simulink model "bramBurst_TransposeMatrix"  (R2021a)
settings: Solver=FixedStepDiscrete  StartTime=0.0  StopTime=44550*Ts  RelTol=1e-3
InitFcn:
  | matched_filter_fft_hdl_init;
model workspace (MAT data in the model file):
  mwTaskManagerKernelLatency = 0
  socvcb = containers.Map
  socvcb.serialization.keys = {12.0018310547, 12.001953125, 12.0020751953, 13.0018310547, 13.001953125, 13.0020751953, 14.0018310547, 14.0020751953, 15.0018310547, 15.0020751953, 15.0133056641, 15.0135498047, 15.0145263672, 15.0153808594, 15.015625, 16.0091552734, 16.0113525391, 16.0115966797, 16.0118408203, 16.0128173828, 16.013671875, 16.0139160156, 16.0141601562, 17.0096435547, 17.0118408203, 17.0146484375, 18.0001220703, 18.0006103516, 19.0001220703, 19.0006103516, 19.0021972656, 19.0023193359, 20.0007324219, 20.0008544922, 30.0006103516, 31.0006103516, 34.0014648438, 35.0014648438, 74.0001220703, 74.0092773438, 74.0178222656, 75.0001220703, 75.0092773438, 75.0178222656, 16098.003418, 20393.0119629, 20461.0002441, 20462.0002441, 21004.0001221, 22191.0001221, 27939.0002441, 29126.0004883, 35663.0014648, 36970.0019531, 48183.0001221, 49370.0001221}
  socvcb.serialization.values : function handle (value not decoded)
  socvcb.serialization.uniformity = 0
  socvcb.serialization.keyType = 'double'
  socvcb.serialization.valueType = 'any'
undefined symbols (not defined in the file or in its folder): columnWindowFun, DTsig_in, DTWindowFun, hdlbramBurst, N1, N2, radarDataCube, Ts
libraries: hdlsllib x35, simulink x11, dsphdlxfrm x1, dsphdlfiltering x1
(part 1 of 2)
settings Model: DataTypeOverride=Off  ExtModeTrigDuration=1  Creator=skuznick  LastModifiedBy=tmealey
settings SolverCC: AlgebraicLoopSolver=TrustRegion  PositivePriorityOrder=on
settings DataIOCC: LimitDataPoints=on  SaveOutput=off  DSMLogging=off  InspectSignalLogs=on  VisualizeSimOutput=off  SaveTime=off
settings OptimizationCC: BlockReduction=off  ConditionallyExecuteInputs=off  DefaultParameterBehavior=Inlined  DefaultUnderspecifiedDataType=single  EnhancedBackFolding=on  PassReuseOutputArgsThreshold=0  EfficientFloat2IntCast=on  MaxStackSize=64  SimCompilerOptimization=on  OptimizeBlockOrder=speed  DifferentSizesBufferReuse=on  OptimizationCustomize=off
settings DebuggingCC: AlgebraicLoopMsg=error  SingleTaskRateTransMsg=error  ParameterPrecisionLossMsg=none  ParameterTunabilityLossMsg=error  FixptConstUnderflowMsg=warning  FixptConstOverflowMsg=warning  AllowSymbolicDim=off  PregeneratedLibrarySubsystemCodeDiagnostic=none  SFUnexpectedBacktrackingDiag=warning  SFNoUnconditionalDefaultTransitionDiag=warning  SFExecutionAtInitializationDiag=none  SFMachineParentedDataDiag=warning  IntegerSaturationMsg=none  ArithmeticOperatorsInVariantConditions=warning
settings HardwareCC: TargetBitPerPointer=64  TargetBitPerSizeT=64  TargetBitPerPtrDiffT=64  TargetLongLongMode=on  TargetIntDivRoundTo=Zero  TargetEndianess=LittleEndian  TargetWordSize=64  TargetHWDeviceType=Custom Processor->MATLAB Host Computer  ProdEqTarget=off  HardwareBoardFeatureSet=SoCBlockset
settings SFSimCC: SimUseLocalCustomCode=off  MATLABDynamicMemAlloc=off  CustomCodeUndefinedFunction=UseInterfaceOnly
settings RTWCC: Description=Generic Real-Time Target  GenerateReport=on  RTWUseLocalCustomCode=off  LaunchReport=on
settings CodeAppCC: ForceParamTrailComments=on  OperatorAnnotations=on
settings GRTTargetCC: TargetLangStandard=C89/C90 (ANSI)
settings ConfigComp: CovMetricSettings=dw  CovSaveCumulativeToWorkspaceVar=on  CovSaveSingleToWorkspaceVar=on  CovExternalEMLEnable=off  CovSFcnEnable=off

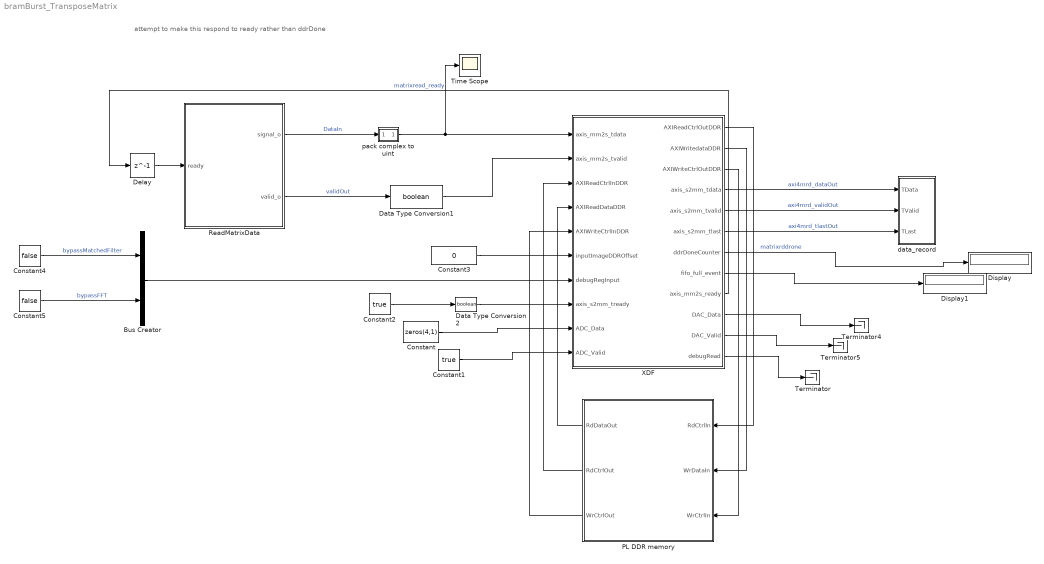
== system bramBurst_TransposeMatrix ==
  note: attempt to make this respond to ready rather than ddrDone
  Bus Creator : BusCreator  Inputs=2
  Constant : Constant  Value=zeros(4,1)  OutDataTypeStr=int16  SampleTime=-1
  Constant1 : Constant  Value=true  OutDataTypeStr=boolean  SampleTime=-1
  Constant2 : Constant  Value=true  SampleTime=-1
  Constant3 : Constant  Value=0  OutDataTypeStr=uint32  SampleTime=-1
  Constant4 : Constant  Value=false  SampleTime=-1
  Constant5 : Constant  Value=false  SampleTime=-1
  Data Type Conversion1 : DataTypeConversion  OutDataTypeStr=boolean
  Data Type Conversion2 : DataTypeConversion  OutDataTypeStr=boolean
  Delay : Delay  DelayLength=1
  Display : Display
  Display1 : Display
  PL DDR memory : Subsystem
  ReadMatrixData : MATLAB Function  TreatAsAtomicUnit=on  SystemSampleTime=Ts  mask{MatrixInput=radarDataCube, ValidGap=0, GapsInMatrix=40, Ts=Ts}
      mask prompts: MatrixInput "Matrix value"; ValidGap "Valid Gap between columns"; GapsInMatrix "Valid Gap between matrix writes"; Ts "Sample Time"
  Terminator : Terminator
  Terminator4 : Terminator
  Terminator5 : Terminator
  Time Scope : Scope
  XDF : Subsystem  TreatAsAtomicUnit=on
  "data_record " : Subsystem
  pack complex to uint : Subsystem
  wires:
  PL DDR memory/2(RdCtrlOut) -> XDF/3(AXIReadCtrlInDDR)
  PL DDR memory/3(WrCtrlOut) -> XDF/5(AXIWriteCtrlInDDR)
  PL DDR memory/1(RdDataOut) -> XDF/4(AXIReadDataDDR)
  XDF/1(AXIReadCtrlOutDDR) -> PL DDR memory/1(RdCtrlIn)
  XDF/2(AXIWritedataDDR) -> PL DDR memory/2(WrDataIn)
  XDF/3(AXIWriteCtrlOutDDR) -> PL DDR memory/3(WrCtrlIn)
  Constant3/1 -> XDF/6(inputImageDDROffset)
  ReadMatrixData/1(signal_o) -> pack complex to uint/1(In1)  "DataIn"
  ReadMatrixData/2(valid_o) -> Data Type Conversion1/1  "validOut"
  pack complex to uint/1(Out1) -> Time Scope/1, XDF/1(axis_mm2s_tdata)
  XDF/4(axis_s2mm_tdata) -> "data_record "/1(TData)  "axi4mrd_dataOut"
  XDF/5(axis_s2mm_tvalid) -> "data_record "/2(TValid)  "axi4mrd_validOut"
  Data Type Conversion1/1 -> XDF/2(axis_mm2s_tvalid)
  XDF/8(fifo_full_event) -> Display1/1
  XDF/7(ddrDoneCounter) -> Display/1  "matrixrddrone"
  XDF/9(axis_mm2s_ready) -> Delay/1  "matrixread_ready"
  Constant/1 -> XDF/9(ADC_Data)
  Constant1/1 -> XDF/10(ADC_Valid)
  XDF/10(DAC_Data) -> Terminator4/1
  XDF/11(DAC_Valid) -> Terminator5/1
  Data Type Conversion2/1 -> XDF/8(axis_s2mm_tready)
  XDF/6(axis_s2mm_tlast) -> "data_record "/3(TLast)  "axi4mrd_tlastOut"
  Constant2/1 -> Data Type Conversion2/1
  Delay/1 -> ReadMatrixData/1(ready)
  Constant4/1 -> Bus Creator/1  "bypassMatchedFilter"
  Constant5/1 -> Bus Creator/2  "bypassFFT"
  Bus Creator/1 -> XDF/7(debugRegInput)
  XDF/12(debugRead) -> Terminator/1

== system bramBurst_TransposeMatrix/PL DDR memory ==
  RdCtrlIn : Inport
  WrDataIn : Inport  Port=2
  WrCtrlIn : Inport  Port=3
  DDR : Subsystem  mask{DDR_SIZE=N1*N2*4*4, INTERFACE_WORD_LENGTH_SELECT=64, INTERFACE_NUM_WORDS=1, INIT_DATA=uint32(1:100), INIT_ADDR=0, BANDWIDTH_DERATING_PCT=10, READ_DOWNTIME=4, toggle=off, save=on, varnameStr='sim_ddr_data'}
      mask prompts: DDR_SIZE "Memory size (bytes):"; INTERFACE_WORD_LENGTH_SELECT "Word length (bits):"; INTERFACE_NUM_WORDS "Number of words:"; INIT_DATA "Initialization data:"; INIT_ADDR "Starting address:"; BANDWIDTH_DERATING_PCT "Bandwidth derating (%)"; READ_DOWNTIME "Read burst downtime (cycles)"; toggle "Read valid toggling"; save "Enabled"; varnameStr "Variable name:"
      mask help: DDR Simulation model
      mask init:
      | blkH = gcbh;
      | 
      | if(DDR_SIZE<=0)
      |     error('Specify a positive value for memory size.' )  
      | end
      | 
      | if( (BANDWIDTH_DERATING_PCT<0) || (BANDWIDTH_DERATING_PCT > 100) )
      |   error('Specify bandwidth derating as a percentage 0-100.' )  
      | end
      | 
      | if (INIT_ADDR < 0)
      |     error('Specify a positive value for starting address.');
      | end
      | 
      | if (mod(INIT_ADDR,4)~=0)
      |     error('Starting address should be multiple of 4 (32-bit aligned).');
      | end
      | 
      | BANDWIDTH_DERATING = BANDWIDTH_DERATING_PCT/100;
      | 
      | INTERFACE_WORD_LENGTH = str2double(get_param(blkH,'INTERFACE_WORD_LENGTH_SELECT'));
      | 
      | DATA_NUM_BYTES = INTERFACE_WORD_LENGTH/8 * INTERFACE_NUM_WORDS;
      | ADDR_BIT_SHIFT = nextpow2(DATA_NUM_BYTES);
      | 
      | switch INTERFACE_WORD_LENGTH
      |     case {8, 16, 32}
      |         INTERFACE_DT = sprintf('uint%d',INTERFACE_WORD_LENGTH);
      |     case {64, 128}
      |         INTERFACE_DT = numerictype(0,INTERFACE_WORD_LENGTH,0);
      | end
      mask TypeOptions INTERFACE_WORD_LENGTH_SELECT: 8 | 16 | 32 | 64 | 128
      mask Callback INTERFACE_WORD_LENGTH_SELECT:
      | blkH = gcbh;
      | mObj  = Simulink.Mask.get(blkH);
      | txtObj = mObj.getDialogControl('INTERFACE_WIDTH_TEXT');
      | 
      | wordLength = str2double(get_param(blkH,'INTERFACE_WORD_LENGTH_SELECT'));
      | numWords = str2double(get_param(blkH,'INTERFACE_NUM_WORDS'));
      | 
      | if isnan(numWords)
      |     valStr = '';
      | else
      |     valStr = num2str(wordLength*numWords);
      | end
      | 
      | txt = sprintf('Total word length:  %s',valStr);
      | 
      | txtObj.Prompt = txt;
      mask Callback INTERFACE_NUM_WORDS:
      | blkH = gcbh;
      | mObj  = Simulink.Mask.get(blkH);
      | txtObj = mObj.getDialogControl('INTERFACE_WIDTH_TEXT');
      | 
      | wordLength = str2double(get_param(blkH,'INTERFACE_WORD_LENGTH_SELECT'));
      | numWords = str2double(get_param(blkH,'INTERFACE_NUM_WORDS'));
      | 
      | if isnan(numWords)
      |     valStr = '';
      | else
      |     valStr = num2str(wordLength*numWords);
      | end
      | 
      | txt = sprintf('Total word length:  %s',valStr);
      | 
      | txtObj.Prompt = txt;
      mask TypeOptions save: Write DDR Data to Workspace/Save to Workspace/save
      mask TypeOptions varnameStr: Write DDR Data to Workspace/Save to Workspace/varnameStr
      mask DialogControl DescGroupVar Prompt: DDR
      mask DialogControl Container6 Prompt: Interface
      mask DialogControl INTERFACE_WIDTH_TEXT Prompt: Total word length:  64
      mask DialogControl DDR_INIT Prompt: Initialization
      mask DialogControl Container7 Prompt: Behavioral
      mask DialogControl BANDWIDTH_DERATING_PCT Tooltip: between 0 to 1
      mask DialogControl Container5 Prompt: Save memory contents at end of simulation
  RdDataOut : Outport  VectorParamsAs1DForOutWhenUnconnected=off
  RdCtrlOut : Outport  Port=2  VectorParamsAs1DForOutWhenUnconnected=off
  WrCtrlOut : Outport  Port=3  VectorParamsAs1DForOutWhenUnconnected=off
  wires:
  WrDataIn/1 -> DDR/2(axi_wr_data)
  RdCtrlIn/1 -> DDR/1(axi_rd_m2s)
  DDR/1(axi_rd_data) -> RdDataOut/1
  DDR/2(axi_rd_s2m) -> RdCtrlOut/1
  WrCtrlIn/1 -> DDR/3(axi_wr_m2s)
  DDR/3(axi_wr_s2m) -> WrCtrlOut/1

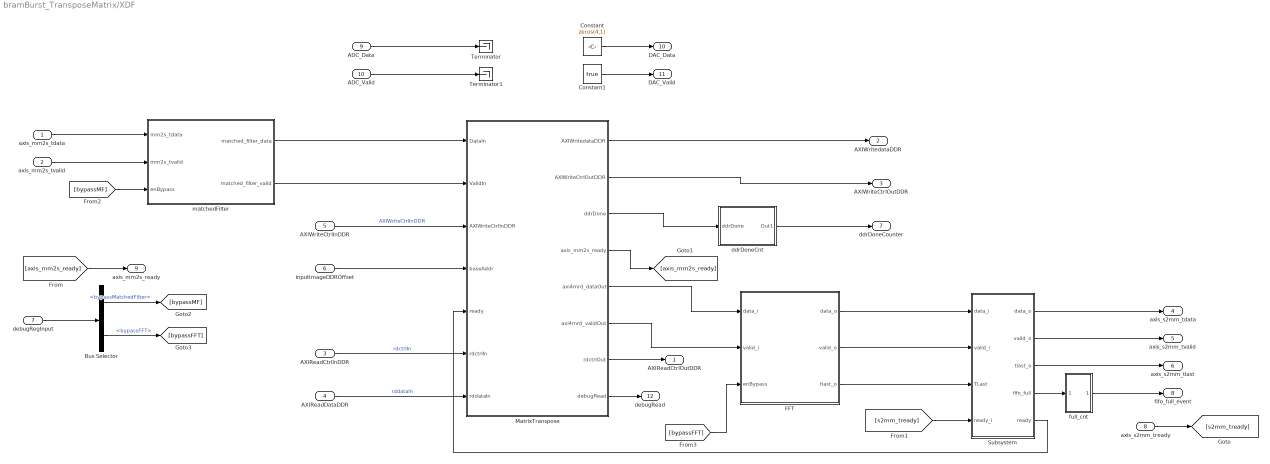
== system bramBurst_TransposeMatrix/XDF ==
  axis_mm2s_tdata : Inport
  axis_mm2s_tvalid : Inport  Port=2
  AXIReadCtrlInDDR : Inport  Port=3
  AXIReadDataDDR : Inport  Port=4
  AXIWriteCtrlInDDR : Inport  Port=5
  inputImageDDROffset : Inport  Port=6
  debugRegInput : Inport  Port=7
  axis_s2mm_tready : Inport  Port=8
  ADC_Data : Inport  Port=9
  ADC_Valid : Inport  Port=10
  Bus Selector : BusSelector  OutputSignals=bypassMatchedFilter,bypassFFT
  Constant : Constant  Value=zeros(4,1)  OutDataTypeStr=int16  SampleTime=-1
  Constant1 : Constant  Value=true  OutDataTypeStr=boolean  SampleTime=-1
  FFT : Subsystem
  MatrixTranspose : Subsystem
  Subsystem : Subsystem
  Terminator : Terminator
  Terminator1 : Terminator
  ddrDoneCnt : Subsystem
  full_cnt : Subsystem
  matchedFilter : Subsystem
  AXIReadCtrlOutDDR : Outport  VectorParamsAs1DForOutWhenUnconnected=off
  AXIWritedataDDR : Outport  Port=2  VectorParamsAs1DForOutWhenUnconnected=off
  AXIWriteCtrlOutDDR : Outport  Port=3  VectorParamsAs1DForOutWhenUnconnected=off
  axis_s2mm_tdata : Outport  Port=4  VectorParamsAs1DForOutWhenUnconnected=off
  axis_s2mm_tvalid : Outport  Port=5
  axis_s2mm_tlast : Outport  Port=6
  ddrDoneCounter : Outport  Port=7
  fifo_full_event : Outport  Port=8
  axis_mm2s_ready : Outport  Port=9
  DAC_Data : Outport  Port=10
  DAC_Valid : Outport  Port=11
  debugRead : Outport  Port=12
  wires:
  axis_mm2s_tvalid/1 -> matchedFilter/2(mm2s_tvalid)
  ADC_Data/1 -> Terminator/1
  ADC_Valid/1 -> Terminator1/1
  Constant/1 -> DAC_Data/1
  Constant1/1 -> DAC_Valid/1
  axis_mm2s_tdata/1 -> matchedFilter/1(mm2s_tdata)
  ddrDoneCnt/1(Out1) -> ddrDoneCounter/1
  Subsystem/1(data_o) -> axis_s2mm_tdata/1
  Subsystem/2(valid_o) -> axis_s2mm_tvalid/1
  Subsystem/3(tlast_o) -> axis_s2mm_tlast/1
  full_cnt/1(Out1) -> fifo_full_event/1
  Subsystem/4(fifo_full) -> full_cnt/1(In1)
  FFT/2(valid_o) -> Subsystem/2(valid_i)
  FFT/3(tlast_o) -> Subsystem/3(TLast)
  FFT/1(data_o) -> Subsystem/1(data_i)
  matchedFilter/1(matched_filter_data) -> MatrixTranspose/1(DataIn)
  matchedFilter/2(matched_filter_valid) -> MatrixTranspose/2(ValidIn)
  AXIWriteCtrlInDDR/1 -> MatrixTranspose/3(AXIWriteCtrlInDDR)  "AXIWriteCtrlInDDR"
  inputImageDDROffset/1 -> MatrixTranspose/4(baseAddr)
  Subsystem/5(ready) -> MatrixTranspose/5(ready)
  AXIReadCtrlInDDR/1 -> MatrixTranspose/6(rdctrlIn)  "rdctrlIn"
  AXIReadDataDDR/1 -> MatrixTranspose/7(rddataIn)  "rddataIn"
  MatrixTranspose/1(AXIWritedataDDR) -> AXIWritedataDDR/1
  MatrixTranspose/2(AXIWriteCtrlOutDDR) -> AXIWriteCtrlOutDDR/1
  MatrixTranspose/3(ddrDone) -> ddrDoneCnt/1(ddrDone)
  MatrixTranspose/4(axis_mm2s_ready) -> [axis_mm2s_ready]
  MatrixTranspose/5(axi4mrd_dataOut) -> FFT/1(data_i)
  MatrixTranspose/6(axi4mrd_validOut) -> FFT/2(valid_i)
  MatrixTranspose/7(rdctrlOut) -> AXIReadCtrlOutDDR/1
  [axis_mm2s_ready] -> axis_mm2s_ready/1
  axis_s2mm_tready/1 -> [s2mm_tready]
  [s2mm_tready] -> Subsystem/4(ready_i)
  debugRegInput/1 -> Bus Selector/1
  Bus Selector/1 -> [bypassMF]  "<bypassMatchedFilter>"
  Bus Selector/2 -> [bypassFFT]  "<bypassFFT>"
  [bypassMF] -> matchedFilter/3(enBypass)
  [bypassFFT] -> FFT/3(enBypass)
  MatrixTranspose/8(debugRead) -> debugRead/1

== system bramBurst_TransposeMatrix/data_record  ==
  TData : Inport
  TValid : Inport  Port=2
  TLast : Inport  Port=3
  Compare To Constant : simulink/Logic and Bit Operations/Compare To Constant  relop=>=  const=N1*N2*1  OutDataTypeStr=boolean
  HDL Counter : hdlsllib/Sources/HDL Counter  CountType=Free running  CountInit=0  CountStep=1  CountMax=25  CountFromType=Initial value  CountFrom=0  CountResetPort=off  CountLoadPort=off  CountEnbPort=on  CountDirPort=off  CountHitOutputPort=off  CountDataType=Unsigned  CountWordLen=32  CountFracLen=0  CountSampTime=1
  Stop Simulation : Stop
  To Workspace : ToWorkspace  VariableName=rdMat  SampleTime=-1
      settings: Save2DSignal=2-D array (concatenate along first dimension)
  To Workspace1 : ToWorkspace  VariableName=rdValid  SampleTime=-1
      settings: Save2DSignal=2-D array (concatenate along first dimension)
  To Workspace2 : ToWorkspace  VariableName=rdTlast  SampleTime=-1
      settings: Save2DSignal=2-D array (concatenate along first dimension)
  "unpack uint to complex " : Subsystem
  wires:
  HDL Counter/1 -> Compare To Constant/1
  Compare To Constant/1 -> Stop Simulation/1
  TValid/1 -> HDL Counter/1, To Workspace1/1
  TData/1 -> "unpack uint to complex "/1(TData)
  TLast/1 -> To Workspace2/1
  "unpack uint to complex "/1(Out1) -> To Workspace/1

== system bramBurst_TransposeMatrix/pack complex to uint ==
  In1 : Inport
  Bit Concat : hdlsllib/Logic and Bit Operations/Bit Concat  numInputs=2
  Bit Concat1 : hdlsllib/Logic and Bit Operations/Bit Concat  Commented=on  numInputs=2
  Complex to Real-Imag : ComplexToRealImag
  Complex to Real-Imag1 : ComplexToRealImag  Commented=on
  Data Type Conversion1 : DataTypeConversion  Commented=on  OutDataTypeStr=fixdt(1,32,28)
  Data Type Conversion2 : DataTypeConversion  OutDataTypeStr=DTsig_in
  Data Type Conversion3 : DataTypeConversion  OutDataTypeStr=uint64  ConvertRealWorld=Stored Integer (SI)
  Out1 : Outport
  wires:
  Complex to Real-Imag/2 -> Bit Concat/2
  Data Type Conversion2/1 -> Complex to Real-Imag/1  "Data"
  Complex to Real-Imag/1 -> Bit Concat/1
  In1/1 -> Data Type Conversion1/1, Data Type Conversion2/1
  Data Type Conversion1/1 -> Complex to Real-Imag1/1  "Data"
  Complex to Real-Imag1/1 -> Bit Concat1/1
  Complex to Real-Imag1/2 -> Bit Concat1/2
  Data Type Conversion3/1 -> Out1/1
  Bit Concat/1 -> Data Type Conversion3/1

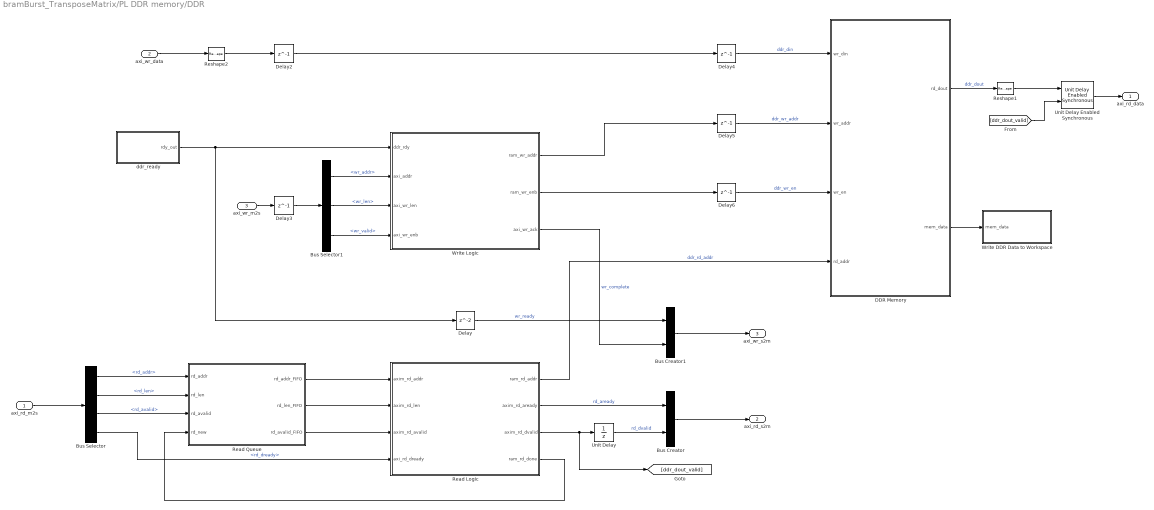
== system bramBurst_TransposeMatrix/PL DDR memory/DDR ==
  axi_rd_m2s : Inport
  axi_wr_data : Inport  Port=2  OutDataTypeStr=INTERFACE_DT  PortDimensions=INTERFACE_NUM_WORDS
  axi_wr_m2s : Inport  Port=3
  Bus Creator : BusCreator  Inputs=2
  Bus Creator1 : BusCreator  Inputs=2  OutDataTypeStr=Bus: BusAXIWriteCtrlS2M  NonVirtualBus=on
  Bus Selector : BusSelector  OutputSignals=rd_addr,rd_len,rd_avalid,rd_dready
  Bus Selector1 : BusSelector  OutputSignals=wr_addr,wr_len,wr_valid
  DDR Memory : MATLAB Function  TreatAsAtomicUnit=on
  Delay : Delay
  Delay{2..6} (5 alike) : Delay  DelayLength=1
  Read Logic : Subsystem
  Read Queue : Subsystem
  Reshape1 : Reshape
  Reshape2 : Reshape
  Unit Delay : UnitDelay  SampleTime=-1  HasFrameUpgradeWarning=on
  Unit Delay Enabled Synchronous : hdlsllib/Discrete/Unit Delay Enabled Synchronous  InitialCondition=0.0  SampleTime=-1
      settings: SourceProductBaseCode=SL
  Write DDR Data to Workspace : Subsystem  TreatAsAtomicUnit=on
  Write Logic : Subsystem
  ddr_ready : Subsystem
  axi_rd_data : Outport  VectorParamsAs1DForOutWhenUnconnected=off
  axi_rd_s2m : Outport  Port=2  VectorParamsAs1DForOutWhenUnconnected=off
  axi_wr_s2m : Outport  Port=3  VectorParamsAs1DForOutWhenUnconnected=off
  wires:
  [ddr_dout_valid] -> Unit Delay Enabled Synchronous/2
  Unit Delay/1 -> Bus Creator/2  "rd_dvalid"
  Unit Delay Enabled Synchronous/1 -> axi_rd_data/1
  Reshape1/1 -> Unit Delay Enabled Synchronous/1
  Reshape2/1 -> Delay2/1
  axi_wr_data/1 -> Reshape2/1
  Read Queue/1(rd_addr_FIFO) -> Read Logic/1(axim_rd_addr)
  Bus Selector/1 -> Read Queue/1(rd_addr)  "<rd_addr>"
  Read Queue/3(rd_avalid_FIFO) -> Read Logic/3(axim_rd_avalid)
  Read Queue/2(rd_len_FIFO) -> Read Logic/2(axim_rd_len)
  Bus Selector/3 -> Read Queue/3(rd_avalid)  "<rd_avalid>"
  Read Logic/4(ram_rd_done) -> Read Queue/4(rd_new)
  Bus Selector/2 -> Read Queue/2(rd_len)  "<rd_len>"
  DDR Memory/2(mem_data) -> Write DDR Data to Workspace/1(mem_data)
  Delay6/1 -> DDR Memory/3(wr_en)  "ddr_wr_en"
  Delay5/1 -> DDR Memory/2(wr_addr)  "ddr_wr_addr"
  Delay4/1 -> DDR Memory/1(wr_din)  "ddr_din"
  axi_rd_m2s/1 -> Bus Selector/1
  Bus Selector/4 -> Read Logic/4(axi_rd_dready)  "<rd_dready>"
  Delay3/1 -> Bus Selector1/1
  Delay2/1 -> Delay4/1
  Delay/1 -> Bus Creator1/1  "wr_ready"
  Write Logic/3(axi_wr_ack) -> Bus Creator1/2  "wr_complete"
  Bus Creator1/1 -> axi_wr_s2m/1
  ddr_ready/1(rdy_out) -> Delay/1, Write Logic/1(ddr_rdy)
  Read Logic/3(axim_rd_dvalid) -> Unit Delay/1, [ddr_dout_valid]
  Bus Creator/1 -> axi_rd_s2m/1
  Read Logic/2(axim_rd_aready) -> Bus Creator/1  "rd_aready"
  Bus Selector1/2 -> Write Logic/3(axi_wr_len)  "<wr_len>"
  Bus Selector1/3 -> Write Logic/4(axi_wr_enb)  "<wr_valid>"
  axi_wr_m2s/1 -> Delay3/1
  Bus Selector1/1 -> Write Logic/2(axi_addr)  "<wr_addr>"
  Write Logic/1(ram_wr_addr) -> Delay5/1
  Read Logic/1(ram_rd_addr) -> DDR Memory/4(rd_addr)  "ddr_rd_addr"
  DDR Memory/1(rd_dout) -> Reshape1/1  "ddr_dout"
  Write Logic/2(ram_wr_enb) -> Delay6/1

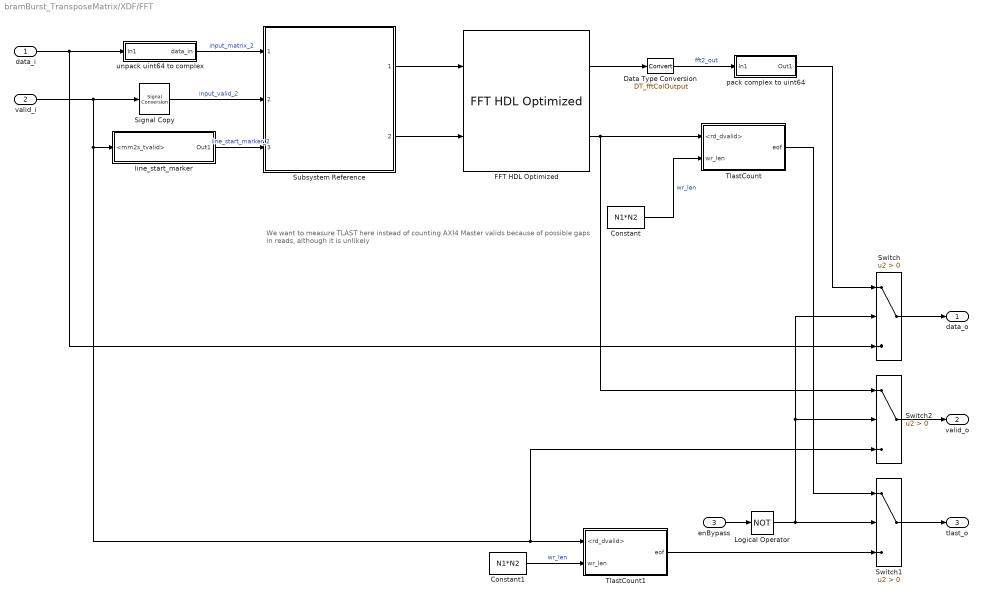
== system bramBurst_TransposeMatrix/XDF/FFT ==
  note: We want to measure TLAST here instead of counting
      | AXI4 Master valids because of possible gaps in reads, although it is unlikely
  data_i : Inport
  valid_i : Inport  Port=2
  enBypass : Inport  Port=3
  Constant : Constant  Value=N1*N2  OutDataTypeStr=uint32  SampleTime=-1
  Constant1 : Constant  Value=N1*N2  OutDataTypeStr=uint32  SampleTime=-1
  Data Type Conversion : DataTypeConversion  OutDataTypeStr=DT_fftColOutput
  FFT HDL Optimized : dsphdlxfrm/FFT HDL Optimized  FFTLength=N2  Architecture=Streaming Radix 2^2  ComplexMultiplication=Use 4 multipliers and 2 adders  BitReversedOutput=off  BitReversedInput=off  Normalize=on  SimulateUsing=Code generation  RoundingMethod=Floor  ResetInputPort=off  StartOutputPort=off  EndOutputPort=off
      settings: SourceProductBaseCode=DS
  Logical Operator : Logic  Operator=NOT  IconShape=distinctive  AllPortsSameDT=off  OutDataTypeStr=boolean
  Signal Copy : SignalConversion  OverrideOpt=off
  Subsystem Reference : Subsystem  ReferencedSubsystem=window_taper  windowFun=fi(columnWindowFun,DTWindowFun)
  Switch : Switch  Criteria=u2 > Threshold
  Switch1 : Switch  Criteria=u2 > Threshold
  Switch2 : Switch  Criteria=u2 > Threshold
  TlastCount : Subsystem
  TlastCount1 : Subsystem
  line_start_marker : Subsystem
  pack complex to uint64 : Subsystem
  "unpack uint64 to complex " : Subsystem
  data_o : Outport
  valid_o : Outport  Port=2
  tlast_o : Outport  Port=3
  wires:
  Data Type Conversion/1 -> pack complex to uint64/1(In1)  "fft2_out"
  Subsystem Reference/2 -> FFT HDL Optimized/2
  Subsystem Reference/1 -> FFT HDL Optimized/1
  "unpack uint64 to complex "/1(data_in) -> Subsystem Reference/1  "input_matrix_2"
  line_start_marker/1(Out1) -> Subsystem Reference/3  "line_start_marker_2"
  FFT HDL Optimized/1 -> Data Type Conversion/1
  Signal Copy/1 -> Subsystem Reference/2  "input_valid_2"
  pack complex to uint64/1(Out1) -> Switch/1
  data_i/1 -> Switch/3, "unpack uint64 to complex "/1(In1)
  enBypass/1 -> Logical Operator/1
  Logical Operator/1 -> Switch2/2, Switch/2, Switch1/2
  Constant/1 -> TlastCount/2(wr_len)  "wr_len"
  FFT HDL Optimized/2 -> TlastCount/1(<rd_dvalid>), Switch2/1
  TlastCount/1(eof) -> Switch1/1
  valid_i/1 -> line_start_marker/1(<mm2s_tvalid>), Switch2/3, TlastCount1/1(<rd_dvalid>), Signal Copy/1
  Constant1/1 -> TlastCount1/2(wr_len)  "wr_len"
  TlastCount1/1(eof) -> Switch1/3
  Switch/1 -> data_o/1
  Switch2/1 -> valid_o/1
  Switch1/1 -> tlast_o/1

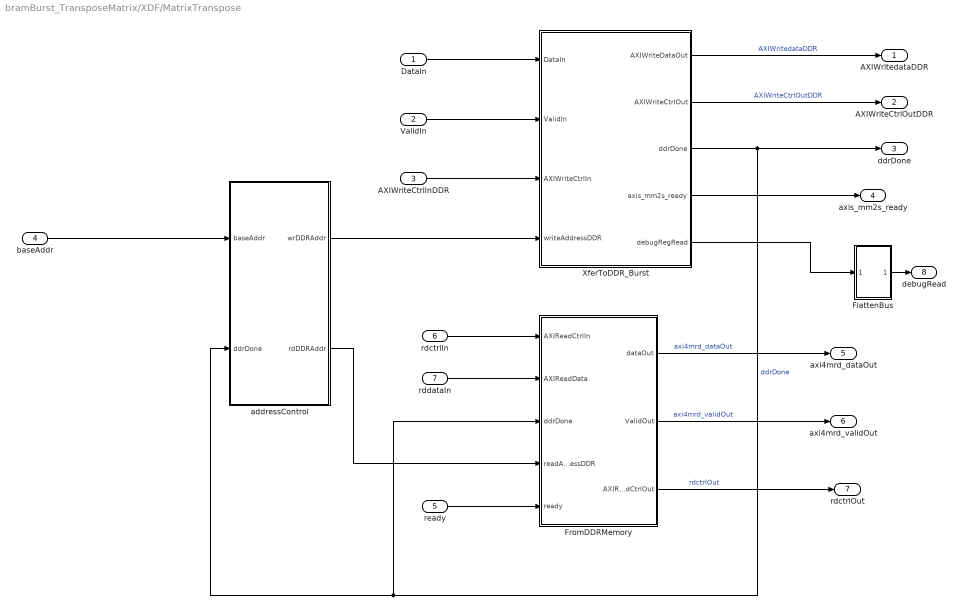
== system bramBurst_TransposeMatrix/XDF/MatrixTranspose ==
  DataIn : Inport
  ValidIn : Inport  Port=2
  AXIWriteCtrlInDDR : Inport  Port=3
  baseAddr : Inport  Port=4
  ready : Inport  Port=5
  rdctrlIn : Inport  Port=6
  rddataIn : Inport  Port=7
  FlattenBus : Subsystem
  FromDDRMemory : Subsystem
  XferToDDR_Burst : Subsystem  VariantControl=XferToDDR_Burst
  addressControl : Subsystem
  AXIWritedataDDR : Outport
  AXIWriteCtrlOutDDR : Outport  Port=2
  ddrDone : Outport  Port=3
  axis_mm2s_ready : Outport  Port=4
  axi4mrd_dataOut : Outport  Port=5
  axi4mrd_validOut : Outport  Port=6
  rdctrlOut : Outport  Port=7
  debugRead : Outport  Port=8
  wires:
  addressControl/2(rdDDRAddr) -> FromDDRMemory/4(readAddressDDR)
  XferToDDR_Burst/3(ddrDone) -> FromDDRMemory/3(ddrDone), addressControl/2(ddrDone), ddrDone/1  "ddrDone"
  FromDDRMemory/1(dataOut) -> axi4mrd_dataOut/1  "axi4mrd_dataOut"
  FromDDRMemory/3(AXIReadCtrlOut) -> rdctrlOut/1  "rdctrlOut"
  addressControl/1(wrDDRAddr) -> XferToDDR_Burst/4(writeAddressDDR)
  DataIn/1 -> XferToDDR_Burst/1(DataIn)
  XferToDDR_Burst/2(AXIWriteCtrlOut) -> AXIWriteCtrlOutDDR/1  "AXIWriteCtrlOutDDR"
  XferToDDR_Burst/1(AXIWriteDataOut) -> AXIWritedataDDR/1  "AXIWritedataDDR"
  rddataIn/1 -> FromDDRMemory/2(AXIReadData)
  XferToDDR_Burst/4(axis_mm2s_ready) -> axis_mm2s_ready/1
  FromDDRMemory/2(ValidOut) -> axi4mrd_validOut/1  "axi4mrd_validOut"
  rdctrlIn/1 -> FromDDRMemory/1(AXIReadCtrlIn)
  baseAddr/1 -> addressControl/1(baseAddr)
  AXIWriteCtrlInDDR/1 -> XferToDDR_Burst/3(AXIWriteCtrlIn)
  ValidIn/1 -> XferToDDR_Burst/2(ValidIn)
  ready/1 -> FromDDRMemory/5(ready)
  XferToDDR_Burst/5(debugRegRead) -> FlattenBus/1(In1)
  FlattenBus/1(Out1) -> debugRead/1

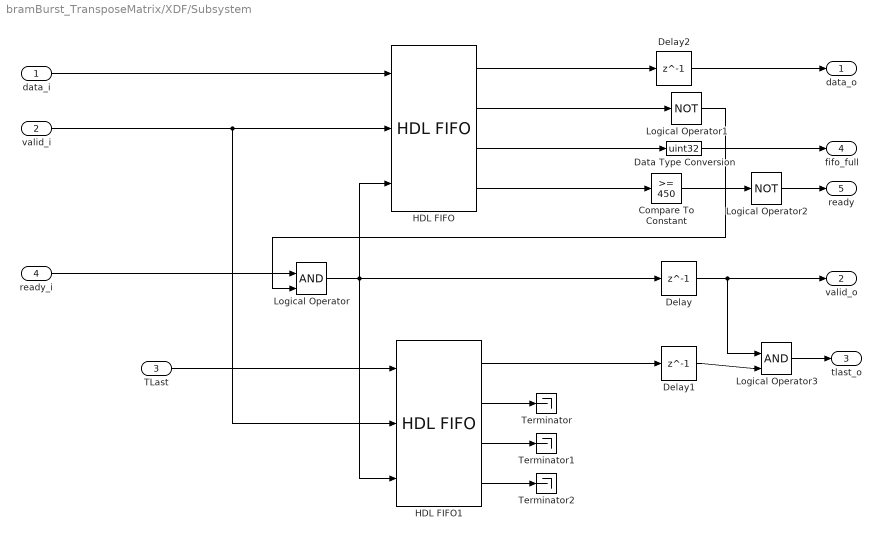
== system bramBurst_TransposeMatrix/XDF/Subsystem ==
  data_i : Inport
  valid_i : Inport  Port=2
  TLast : Inport  Port=3
  ready_i : Inport  Port=4
  Compare To Constant : simulink/Logic and Bit Operations/Compare To Constant  relop=>=  const=450  OutDataTypeStr=boolean
  Data Type Conversion : DataTypeConversion  OutDataTypeStr=uint32
  Delay : Delay  DelayLength=1
  Delay1 : Delay  DelayLength=1
  Delay2 : Delay  DelayLength=1
  HDL FIFO : hdlsllib/HDL RAMs/HDL FIFO  fifo_size=512  mode=FWFT  ratio=1  push_msg=Warning  pop_msg=Warning  show_empty=on  show_full=on  show_num=on  LabelModeActiveChoice_Mode=FWFT
      settings: SourceProductBaseCode=SL
  HDL FIFO1 : hdlsllib/HDL RAMs/HDL FIFO  fifo_size=512  mode=FWFT  ratio=1  push_msg=Warning  pop_msg=Warning  show_empty=on  show_full=on  show_num=on  LabelModeActiveChoice_Mode=FWFT
      settings: SourceProductBaseCode=SL
  Logical Operator : Logic  IconShape=distinctive  AllPortsSameDT=off  OutDataTypeStr=boolean
  Logical Operator1 : Logic  Operator=NOT  IconShape=distinctive  AllPortsSameDT=off  OutDataTypeStr=boolean
  Logical Operator2 : Logic  Operator=NOT  IconShape=distinctive  AllPortsSameDT=off  OutDataTypeStr=boolean
  Logical Operator3 : Logic  IconShape=distinctive  AllPortsSameDT=off  OutDataTypeStr=boolean
  Terminator : Terminator
  Terminator1 : Terminator
  Terminator2 : Terminator
  data_o : Outport
  valid_o : Outport  Port=2
  tlast_o : Outport  Port=3
  fifo_full : Outport  Port=4
  ready : Outport  Port=5
  wires:
  valid_i/1 -> HDL FIFO1/2, HDL FIFO/2
  Logical Operator1/1 -> Logical Operator/2
  HDL FIFO/4 -> Compare To Constant/1
  HDL FIFO/1 -> Delay2/1
  Logical Operator/1 -> HDL FIFO1/3, Delay/1, HDL FIFO/3
  HDL FIFO/3 -> Data Type Conversion/1
  Delay2/1 -> data_o/1
  HDL FIFO/2 -> Logical Operator1/1
  data_i/1 -> HDL FIFO/1
  Data Type Conversion/1 -> fifo_full/1
  ready_i/1 -> Logical Operator/1
  Delay/1 -> Logical Operator3/1, valid_o/1
  Compare To Constant/1 -> Logical Operator2/1
  Logical Operator2/1 -> ready/1
  TLast/1 -> HDL FIFO1/1
  HDL FIFO1/2 -> Terminator/1
  HDL FIFO1/3 -> Terminator1/1
  HDL FIFO1/4 -> Terminator2/1
  Delay1/1 -> Logical Operator3/2
  HDL FIFO1/1 -> Delay1/1
  Logical Operator3/1 -> tlast_o/1

== system bramBurst_TransposeMatrix/XDF/ddrDoneCnt ==
  ddrDone : Inport
  Add : Sum  AccumDataTypeStr=uint32
  Data Type Conversion : DataTypeConversion  OutDataTypeStr=uint32
  Delay1 : Delay  DelayLength=1
  Out1 : Outport
  wires:
  ddrDone/1 -> Data Type Conversion/1
  Delay1/1 -> Out1/1, Add/2
  Add/1 -> Delay1/1
  Data Type Conversion/1 -> Add/1

== system bramBurst_TransposeMatrix/XDF/full_cnt ==
  In1 : Inport
  Add : Sum  AccumDataTypeStr=uint32
  Delay1 : Delay  DelayLength=1
  Out1 : Outport
  wires:
  In1/1 -> Add/1
  Delay1/1 -> Out1/1, Add/2
  Add/1 -> Delay1/1

== system bramBurst_TransposeMatrix/XDF/matchedFilter ==
  mm2s_tdata : Inport
  mm2s_tvalid : Inport  Port=2
  enBypass : Inport  Port=3
  Data Type Conversion1 : DataTypeConversion  OutDataTypeStr=int64  ConvertRealWorld=Stored Integer (SI)
  Data Type Conversion2 : DataTypeConversion  OutDataTypeStr=DTTransposeInOut
  DiscreteFIR_DirectFormTransposed : dsphdlfiltering/Discrete FIR Filter HDL Optimized  NumeratorSource=Property  Numerator=matchingCoeff.'  NumeratorPrototype=[]  FilterStructure=Direct form transposed  SerializationOption=Minimum number of cycles between valid input samples  NumberOfCycles=2  NumberOfMultipliers=2  SimulateUsing=Code generation  roundingMode=Floor  overflowMode=off  CoefficientsDataTypeStr=Inherit: Same word length as input  CoefficientsMin=[]  CoefficientsMax=[]  OutputMin=[]  OutputMax=[]  ResetInputPort=off  HDLGlobalReset=off
      settings: SourceProductBaseCode=DS
  Logical Operator : Logic  Operator=NOT  IconShape=distinctive  AllPortsSameDT=off  OutDataTypeStr=boolean
  Switch : Switch  Criteria=u2 > Threshold
  Switch1 : Switch  Criteria=u2 > Threshold
  pack complex to uint1 : Subsystem
  "unpack uint to DTsig_in " : Subsystem
  matched_filter_data : Outport
  matched_filter_valid : Outport  Port=2
  wires:
  "unpack uint to DTsig_in "/1(Out1) -> DiscreteFIR_DirectFormTransposed/1  "matched_filter_data_in"
  mm2s_tdata/1 -> "unpack uint to DTsig_in "/1(In1), Data Type Conversion1/1
  mm2s_tvalid/1 -> DiscreteFIR_DirectFormTransposed/2, Switch1/3  "matched_filter_valid_in"
  enBypass/1 -> Logical Operator/1
  Logical Operator/1 -> Switch1/2, Switch/2
  Switch1/1 -> matched_filter_valid/1
  Data Type Conversion1/1 -> Switch/3
  Switch/1 -> matched_filter_data/1
  Data Type Conversion2/1 -> pack complex to uint1/1(In1)
  pack complex to uint1/1(matched_filter_data) -> Switch/1  "matched_filter_data"
  DiscreteFIR_DirectFormTransposed/2 -> Switch1/1  "matched_filter_valid_out"
  DiscreteFIR_DirectFormTransposed/1 -> Data Type Conversion2/1  "matched_filter_data_out"

== system bramBurst_TransposeMatrix/data_record /unpack uint to complex  ==
  TData : Inport
  Bit Slice : hdlsllib/Logic and Bit Operations/Bit Slice  lidx=63  ridx=32
      settings: SourceProductBaseCode=SL
  Bit Slice1 : hdlsllib/Logic and Bit Operations/Bit Slice  lidx=31  ridx=0
      settings: SourceProductBaseCode=SL
  Bit Slice2 : hdlsllib/Logic and Bit Operations/Bit Slice  Commented=on  lidx=39  ridx=20
      settings: SourceProductBaseCode=SL
  Bit Slice3 : hdlsllib/Logic and Bit Operations/Bit Slice  Commented=on  lidx=19  ridx=0
      settings: SourceProductBaseCode=SL
  Data Type Conversion : DataTypeConversion  Commented=on  OutDataTypeStr=fixdt(1,20,18)  ConvertRealWorld=Stored Integer (SI)
  Data Type Conversion1 : DataTypeConversion  OutDataTypeStr=double
  Data Type Conversion2 : DataTypeConversion  OutDataTypeStr=DT_fftColOutput  ConvertRealWorld=Stored Integer (SI)
  Real-Imag to Complex : RealImagToComplex
  Real-Imag to Complex1 : RealImagToComplex  Commented=on
  Out1 : Outport
  wires:
  Bit Slice1/1 -> Real-Imag to Complex/2
  Bit Slice/1 -> Real-Imag to Complex/1
  TData/1 -> Bit Slice3/1, Bit Slice2/1, Bit Slice1/1, Bit Slice/1
  Bit Slice2/1 -> Real-Imag to Complex1/1
  Bit Slice3/1 -> Real-Imag to Complex1/2
  Real-Imag to Complex1/1 -> Data Type Conversion/1
  Data Type Conversion1/1 -> Out1/1
  Real-Imag to Complex/1 -> Data Type Conversion2/1
  Data Type Conversion2/1 -> Data Type Conversion1/1

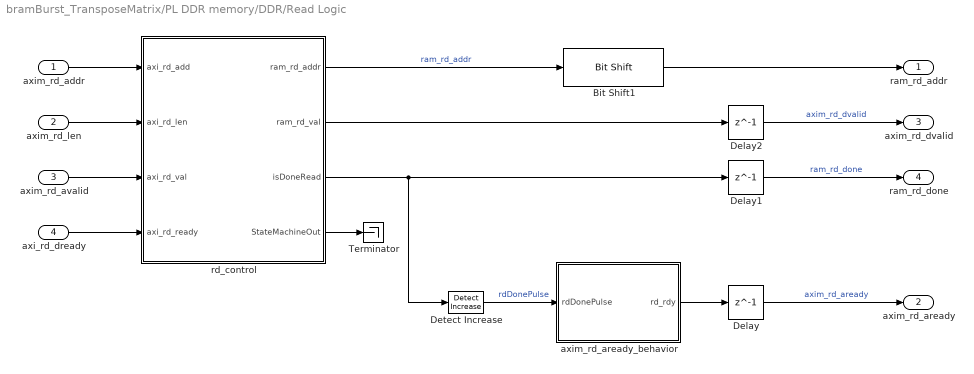
== system bramBurst_TransposeMatrix/PL DDR memory/DDR/Read Logic ==
  axim_rd_addr : Inport
  axim_rd_len : Inport  Port=2
  axim_rd_avalid : Inport  Port=3
  axi_rd_dready : Inport  Port=4
  Bit Shift1 : hdlsllib/Logic and Bit Operations/Bit Shift  mode=Shift Left Logical  N=ADDR_BIT_SHIFT
  Delay : Delay  DelayLength=1
  Delay1 : Delay  DelayLength=1
  Delay2 : Delay  DelayLength=1
  Detect Increase : simulink/Logic and Bit Operations/Detect Increase  vinit=0.0  OutDataTypeStr=boolean
  Terminator : Terminator
  axim_rd_aready_behavior : MATLAB Function  TreatAsAtomicUnit=on
  rd_control : MATLAB Function  TreatAsAtomicUnit=on
  ram_rd_addr : Outport  VectorParamsAs1DForOutWhenUnconnected=off
  axim_rd_aready : Outport  Port=2  VectorParamsAs1DForOutWhenUnconnected=off
  axim_rd_dvalid : Outport  Port=3  VectorParamsAs1DForOutWhenUnconnected=off
  ram_rd_done : Outport  Port=4  VectorParamsAs1DForOutWhenUnconnected=off
  wires:
  Bit Shift1/1 -> ram_rd_addr/1
  axim_rd_aready_behavior/1(rd_rdy) -> Delay/1
  Detect Increase/1 -> axim_rd_aready_behavior/1(rdDonePulse)  "rdDonePulse"
  rd_control/4(StateMachineOut) -> Terminator/1
  Delay1/1 -> ram_rd_done/1  "ram_rd_done"
  rd_control/3(isDoneRead) -> Delay1/1, Detect Increase/1
  rd_control/2(ram_rd_val) -> Delay2/1
  axim_rd_len/1 -> rd_control/2(axi_rd_len)
  Delay/1 -> axim_rd_aready/1  "axim_rd_aready"
  Delay2/1 -> axim_rd_dvalid/1  "axim_rd_dvalid"
  axi_rd_dready/1 -> rd_control/4(axi_rd_ready)
  rd_control/1(ram_rd_addr) -> Bit Shift1/1  "ram_rd_addr"
  axim_rd_avalid/1 -> rd_control/3(axi_rd_val)
  axim_rd_addr/1 -> rd_control/1(axi_rd_add)

== system bramBurst_TransposeMatrix/PL DDR memory/DDR/Read Queue ==
  rd_addr : Inport
  rd_len : Inport  Port=2
  rd_avalid : Inport  Port=3
  rd_new : Inport  Port=4
  Data Type Conversion1 : DataTypeConversion  OutDataTypeStr=uint32
  HDL FIFO1 : hdlsllib/HDL RAMs/HDL FIFO  fifo_size=4  mode=FWFT  ratio=1  push_msg=Warning  pop_msg=Warning  show_empty=on  show_full=off  show_num=off  LabelModeActiveChoice_Mode=FWFT
      settings: SourceProductBaseCode=SL
  HDL FIFO2 : hdlsllib/HDL RAMs/HDL FIFO  fifo_size=4  mode=FWFT  ratio=1  push_msg=Warning  pop_msg=Warning  show_empty=off  show_full=off  show_num=off  LabelModeActiveChoice_Mode=FWFT
      settings: SourceProductBaseCode=SL
  Logical Operator : Logic  Operator=NOT  IconShape=distinctive  AllPortsSameDT=off  OutDataTypeStr=boolean
  Logical Operator1 : Logic  IconShape=distinctive  AllPortsSameDT=off  OutDataTypeStr=boolean
  rd_addr_FIFO : Outport
  rd_len_FIFO : Outport  Port=2
  rd_avalid_FIFO : Outport  Port=3
  wires:
  rd_new/1 -> Logical Operator1/1
  HDL FIFO2/1 -> rd_addr_FIFO/1
  rd_addr/1 -> HDL FIFO2/1
  rd_len/1 -> HDL FIFO1/1
  rd_avalid/1 -> HDL FIFO1/2, HDL FIFO2/2
  Data Type Conversion1/1 -> rd_len_FIFO/1
  Logical Operator/1 -> Logical Operator1/2
  Logical Operator1/1 -> rd_avalid_FIFO/1, HDL FIFO1/3, HDL FIFO2/3
  HDL FIFO1/2 -> Logical Operator/1
  HDL FIFO1/1 -> Data Type Conversion1/1

== system bramBurst_TransposeMatrix/PL DDR memory/DDR/Write DDR Data to Workspace ==
  mem_data : Inport
  Event Listener : EventListener  DisableCoverage=on  EventType=Terminate  EventName=reset
  Save to Workspace : MATLAB Function  TreatAsAtomicUnit=on  mask{varnameStr=varnameStr, save=on}
      mask prompts: varnameStr "Variable name:"; save "Enabled?"
      mask init:
      | varname = uint8(varnameStr);
  wires:
  mem_data/1 -> Save to Workspace/1(data)

== system bramBurst_TransposeMatrix/PL DDR memory/DDR/Write Logic ==
  ddr_rdy : Inport
  axi_addr : Inport  Port=2
  axi_wr_len : Inport  Port=3
  axi_wr_enb : Inport  Port=4
  Add : Sum  AccumDataTypeStr=uint32
  Bit Shift1 : hdlsllib/Logic and Bit Operations/Bit Shift  mode=Shift Left Logical  N=ADDR_BIT_SHIFT
  Logical Operator : Logic  Operator=OR  IconShape=distinctive  AllPortsSameDT=off  OutDataTypeStr=boolean
  Wr_control : Subsystem
  ddr_ack_d1 : Delay  DelayLength=1
  ddr_reday_d1 : Delay  DelayLength=1
  ddr_reday_d6 : Delay  DelayLength=4
  ram_wr_addr : Outport  VectorParamsAs1DForOutWhenUnconnected=off
  ram_wr_enb : Outport  Port=2  VectorParamsAs1DForOutWhenUnconnected=off
  axi_wr_ack : Outport  Port=3  VectorParamsAs1DForOutWhenUnconnected=off
  wires:
  Bit Shift1/1 -> Add/2
  Logical Operator/1 -> Wr_control/1(ddr_wr_rdy)
  ddr_reday_d1/1 -> Logical Operator/1
  axi_addr/1 -> Add/1
  ddr_ack_d1/1 -> axi_wr_ack/1
  ddr_reday_d6/1 -> Logical Operator/2, ddr_reday_d1/1
  Wr_control/3(ram_addr) -> Bit Shift1/1
  Add/1 -> ram_wr_addr/1
  Wr_control/2(axim_ack) -> ddr_ack_d1/1
  axi_wr_enb/1 -> Wr_control/2(wr_enb)
  ddr_rdy/1 -> ddr_reday_d6/1
  axi_wr_len/1 -> Wr_control/3(wr_len)
  Wr_control/1(valAddEnb) -> ram_wr_enb/1

== system bramBurst_TransposeMatrix/PL DDR memory/DDR/ddr_ready ==
  READY generation : MATLAB Function  TreatAsAtomicUnit=on
  rdy_out : Outport  VectorParamsAs1DForOutWhenUnconnected=off
  wires:
  READY generation/1(ready) -> rdy_out/1

== system bramBurst_TransposeMatrix/XDF/FFT/TlastCount ==
  <rd_dvalid> : Inport
  wr_len : Inport  Port=2
  Decrement Real World : simulink/Additional Math & Discrete/Additional Math: Increment - Decrement/Decrement Real World
      settings: SourceProductBaseCode=SL
  HDL Counter : hdlsllib/Sources/HDL Counter  CountType=Free running  CountInit=0  CountStep=1  CountMax=25  CountFromType=Initial value  CountFrom=0  CountResetPort=on  CountLoadPort=off  CountEnbPort=on  CountDirPort=off  CountHitOutputPort=off  CountDataType=Unsigned  CountWordLen=32  CountFracLen=0  CountSampTime=1
  Relational Operator : RelationalOperator  Operator===  OutDataTypeStr=boolean  RndMeth=Simplest
  eof : Outport
  wires:
  wr_len/1 -> Decrement Real World/1
  <rd_dvalid>/1 -> HDL Counter/2
  HDL Counter/1 -> Relational Operator/1
  Relational Operator/1 -> HDL Counter/1, eof/1
  Decrement Real World/1 -> Relational Operator/2

== system bramBurst_TransposeMatrix/XDF/FFT/TlastCount1 ==
  <rd_dvalid> : Inport
  wr_len : Inport  Port=2
  Decrement Real World : simulink/Additional Math & Discrete/Additional Math: Increment - Decrement/Decrement Real World
      settings: SourceProductBaseCode=SL
  HDL Counter : hdlsllib/Sources/HDL Counter  CountType=Free running  CountInit=0  CountStep=1  CountMax=25  CountFromType=Initial value  CountFrom=0  CountResetPort=on  CountLoadPort=off  CountEnbPort=on  CountDirPort=off  CountHitOutputPort=off  CountDataType=Unsigned  CountWordLen=32  CountFracLen=0  CountSampTime=1
  Relational Operator : RelationalOperator  Operator===  OutDataTypeStr=boolean  RndMeth=Simplest
  eof : Outport
  wires:
  wr_len/1 -> Decrement Real World/1
  <rd_dvalid>/1 -> HDL Counter/2
  HDL Counter/1 -> Relational Operator/1
  Relational Operator/1 -> HDL Counter/1, eof/1
  Decrement Real World/1 -> Relational Operator/2

== system bramBurst_TransposeMatrix/XDF/FFT/line_start_marker ==
  <mm2s_tvalid> : Inport
  AND : Logic  IconShape=distinctive  AllPortsSameDT=off  OutDataTypeStr=boolean
  Compare To Constant : simulink/Logic and Bit Operations/Compare To Constant  relop===  const=0  OutDataTypeStr=boolean
  HDL Counter : hdlsllib/Sources/HDL Counter  CountType=Count limited  CountInit=0  CountStep=1  CountMax=N2-1  CountFromType=Initial value  CountFrom=0  CountResetPort=off  CountLoadPort=off  CountEnbPort=on  CountDirPort=off  CountHitOutputPort=off  CountDataType=Unsigned  CountWordLen=16  CountFracLen=0  CountSampTime=1
  Out1 : Outport
  wires:
  <mm2s_tvalid>/1 -> AND/1, HDL Counter/1
  HDL Counter/1 -> Compare To Constant/1
  Compare To Constant/1 -> AND/2
  AND/1 -> Out1/1

== system bramBurst_TransposeMatrix/XDF/FFT/pack complex to uint64 ==
  In1 : Inport
  Bit Concat : hdlsllib/Logic and Bit Operations/Bit Concat  numInputs=2
  Complex to Real-Imag : ComplexToRealImag
  Out1 : Outport
  wires:
  Complex to Real-Imag/2 -> Bit Concat/2
  In1/1 -> Complex to Real-Imag/1  "Data"
  Complex to Real-Imag/1 -> Bit Concat/1
  Bit Concat/1 -> Out1/1

== system bramBurst_TransposeMatrix/XDF/FFT/unpack uint64 to complex  ==
  In1 : Inport
  Bit Slice : hdlsllib/Logic and Bit Operations/Bit Slice  lidx=63  ridx=32
      settings: SourceProductBaseCode=SL
  Bit Slice1 : hdlsllib/Logic and Bit Operations/Bit Slice  lidx=31  ridx=0
      settings: SourceProductBaseCode=SL
  Data Type Conversion : DataTypeConversion  OutDataTypeStr=DTTransposeInOut  ConvertRealWorld=Stored Integer (SI)
  Real-Imag to Complex : RealImagToComplex
  data_in : Outport
  wires:
  Bit Slice1/1 -> Real-Imag to Complex/2
  Bit Slice/1 -> Real-Imag to Complex/1
  Data Type Conversion/1 -> data_in/1
  Real-Imag to Complex/1 -> Data Type Conversion/1
  In1/1 -> Bit Slice1/1, Bit Slice/1

== system bramBurst_TransposeMatrix/XDF/MatrixTranspose/FlattenBus ==
  In1 : Inport
  Bus Creator : BusCreator  Inputs=9
  Bus Selector : BusSelector  OutputSignals=DataWrLogicDebug.wr_complete_counter,DataWrLogicDebug.bankCompleteCounter,DataWrLogicDebug.FIFO_back_pressure_applied,DataWrLogicDebug.CountWriteValids,DataWrLogicDebug.FSM_read,FIFODebugReg.FIFO_Full_eventCount,FIFODebugReg.lostSampleCount,FIFODebugReg.axis_mm2s_backpressure_cnt,FIFODebugReg.FIFO_Output_valid_counter
  Signal Conversion{,1..8} (9 alike) : SignalConversion  OverrideOpt=off
  Out1 : Outport
  wires:
  In1/1 -> Bus Selector/1
  Bus Selector/9 -> Signal Conversion8/1  "<FIFO_Output_valid_counter>"
  Bus Selector/8 -> Signal Conversion7/1  "<axis_mm2s_backpressure_cnt>"
  Bus Selector/7 -> Signal Conversion6/1  "<lostSampleCount>"
  Bus Selector/6 -> Signal Conversion5/1  "<FIFO_Full_eventCount>"
  Bus Selector/5 -> Signal Conversion4/1  "<FSM_read>"
  Bus Selector/4 -> Signal Conversion3/1  "<CountWriteValids>"
  Bus Selector/3 -> Signal Conversion2/1  "<FIFO_back_pressure_applied>"
  Bus Selector/2 -> Signal Conversion1/1  "<bankCompleteCounter>"
  Bus Selector/1 -> Signal Conversion/1  "<wr_complete_counter>"
  Bus Creator/1 -> Out1/1
  Signal Conversion/1 -> Bus Creator/1  "AXI4M_WrValidCnt"
  Signal Conversion1/1 -> Bus Creator/2  "BRAM_FSM_BankRdCompleteCnt"
  Signal Conversion2/1 -> Bus Creator/3  "BRAM_FSM_StoppingFIFO_Counter"
  Signal Conversion3/1 -> Bus Creator/4  "AXI4M_WriteCounter"
  Signal Conversion4/1 -> Bus Creator/5  "BRAM_FSM_Concat"
  Signal Conversion5/1 -> Bus Creator/6  "FIFO_FullEventCount"
  Signal Conversion6/1 -> Bus Creator/7  "FIFO_LostSampleCount"
  Signal Conversion7/1 -> Bus Creator/8  "FIFO_BackPressureAppliedOnMM2S"
  Signal Conversion8/1 -> Bus Creator/9  "FIFO_ValidWriteCount"

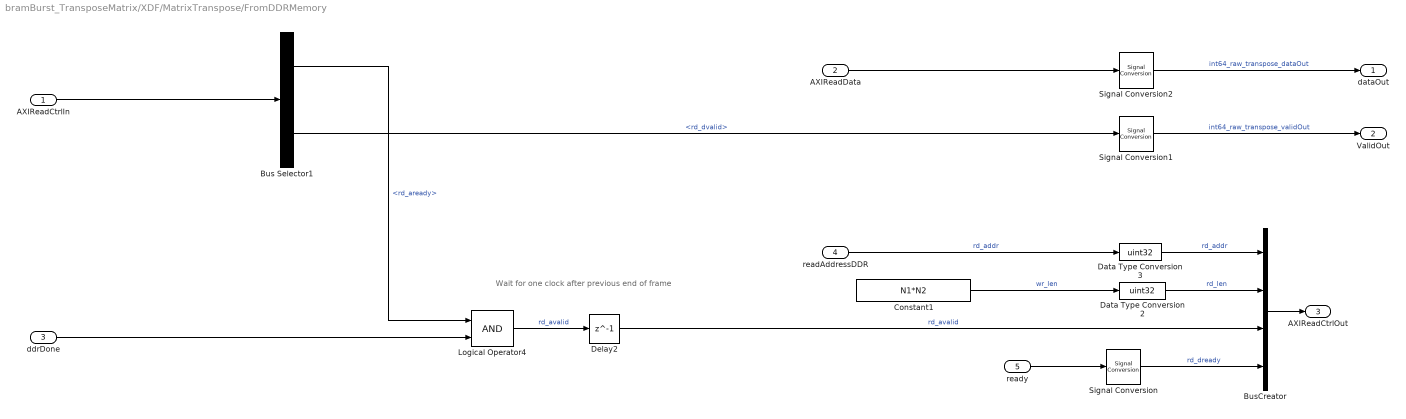
== system bramBurst_TransposeMatrix/XDF/MatrixTranspose/FromDDRMemory ==
  note: Wait for one clock after previous end of frame
  AXIReadCtrlIn : Inport
  AXIReadData : Inport  Port=2
  ddrDone : Inport  Port=3
  readAddressDDR : Inport  Port=4
  ready : Inport  Port=5
  Bus Selector1 : BusSelector  OutputSignals=rd_aready,rd_dvalid
  BusCreator : BusCreator  Inputs=4
  Constant1 : Constant  Value=N1*N2  OutDataTypeStr=uint32  SampleTime=-1
  Data Type Conversion2 : DataTypeConversion  OutDataTypeStr=uint32
  Data Type Conversion3 : DataTypeConversion  OutDataTypeStr=uint32
  Delay2 : Delay  DelayLength=1  InitialCondition=0
  Logical Operator4 : Logic  IconShape=distinctive  AllPortsSameDT=off  OutDataTypeStr=boolean
  Signal Conversion : SignalConversion  OverrideOpt=off
  Signal Conversion1 : SignalConversion  OverrideOpt=off
  Signal Conversion2 : SignalConversion  OverrideOpt=off
  dataOut : Outport  VectorParamsAs1DForOutWhenUnconnected=off
  ValidOut : Outport  Port=2
  AXIReadCtrlOut : Outport  Port=3  VectorParamsAs1DForOutWhenUnconnected=off
  wires:
  Delay2/1 -> BusCreator/3  "rd_avalid"
  Signal Conversion/1 -> BusCreator/4  "rd_dready"
  Bus Selector1/1 -> Logical Operator4/1  "<rd_aready>"
  BusCreator/1 -> AXIReadCtrlOut/1
  Bus Selector1/2 -> Signal Conversion1/1  "<rd_dvalid>"
  Logical Operator4/1 -> Delay2/1  "rd_avalid"
  AXIReadData/1 -> Signal Conversion2/1
  Constant1/1 -> Data Type Conversion2/1  "wr_len"
  Data Type Conversion2/1 -> BusCreator/2  "rd_len"
  AXIReadCtrlIn/1 -> Bus Selector1/1
  Data Type Conversion3/1 -> BusCreator/1  "rd_addr"
  readAddressDDR/1 -> Data Type Conversion3/1  "rd_addr"
  ddrDone/1 -> Logical Operator4/2
  ready/1 -> Signal Conversion/1
  Signal Conversion1/1 -> ValidOut/1  "int64_raw_transpose_validOut"
  Signal Conversion2/1 -> dataOut/1  "int64_raw_transpose_dataOut"

== system bramBurst_TransposeMatrix/XDF/MatrixTranspose/XferToDDR_Burst ==
  DataIn : Inport
  ValidIn : Inport  Port=2
  AXIWriteCtrlIn : Inport  Port=3
  writeAddressDDR : Inport  Port=4
  BackpressureFIFO : Subsystem
  Bus Creator : BusCreator  Inputs=2
  DataWrLogic : Subsystem
  Delay4 : Delay  DelayLength=1
  AXIWriteDataOut : Outport
  AXIWriteCtrlOut : Outport  Port=2
  ddrDone : Outport  Port=3
  axis_mm2s_ready : Outport  Port=4
  debugRegRead : Outport  Port=5
  wires:
  BackpressureFIFO/2(valid_o) -> DataWrLogic/2(ValidIn)
  BackpressureFIFO/1(data_o) -> DataWrLogic/1(DataIn)
  DataWrLogic/1(data) -> AXIWriteDataOut/1  "WrData_s2m"
  DataWrLogic/2(WrCtrlOut) -> AXIWriteCtrlOut/1
  AXIWriteCtrlIn/1 -> DataWrLogic/3(WrCtrlIn)
  DataWrLogic/3(matrix_wr_done) -> ddrDone/1
  writeAddressDDR/1 -> DataWrLogic/4(baseAddr)
  BackpressureFIFO/3(axis_ready) -> axis_mm2s_ready/1
  Delay4/1 -> BackpressureFIFO/3(ready)
  DataWrLogic/4(axis_mm2s_ready) -> Delay4/1
  DataIn/1 -> BackpressureFIFO/1(data_i)
  ValidIn/1 -> BackpressureFIFO/2(valid_i)
  DataWrLogic/5(debugMeasure) -> Bus Creator/1  "DataWrLogicDebug"
  BackpressureFIFO/4(FIFO_Debug) -> Bus Creator/2  "FIFODebugReg"
  Bus Creator/1 -> debugRegRead/1

== system bramBurst_TransposeMatrix/XDF/MatrixTranspose/addressControl ==
  baseAddr : Inport
  ddrDone : Inport  Port=2
  DDRbaseAddrCalc : Subsystem
  ping_pong : Subsystem
  wrDDRAddr : Outport
  rdDDRAddr : Outport  Port=2
  wires:
  ping_pong/1(ddrBank) -> DDRbaseAddrCalc/2(ddrBank)  "bankReadDDR"
  ddrDone/1 -> ping_pong/1(ddrDone)
  baseAddr/1 -> DDRbaseAddrCalc/1(baseAddr)
  DDRbaseAddrCalc/1(ddrWrAddr) -> wrDDRAddr/1  "wrDDRAddr"
  DDRbaseAddrCalc/2(ddrRdAddr) -> rdDDRAddr/1  "rdDDRAddr"

== system bramBurst_TransposeMatrix/XDF/matchedFilter/pack complex to uint1 ==
  In1 : Inport
  Bit Concat : hdlsllib/Logic and Bit Operations/Bit Concat  numInputs=2
  Complex to Real-Imag : ComplexToRealImag
  matched_filter_data : Outport
  wires:
  Complex to Real-Imag/2 -> Bit Concat/2
  In1/1 -> Complex to Real-Imag/1  "Data"
  Complex to Real-Imag/1 -> Bit Concat/1
  Bit Concat/1 -> matched_filter_data/1

== system bramBurst_TransposeMatrix/XDF/matchedFilter/unpack uint to DTsig_in  ==
  In1 : Inport
  Bit Slice : hdlsllib/Logic and Bit Operations/Bit Slice  lidx=DTsig_in.WordLength*2 -1  ridx=DTsig_in.WordLength
      settings: SourceProductBaseCode=SL
  Bit Slice1 : hdlsllib/Logic and Bit Operations/Bit Slice  lidx=DTsig_in.WordLength - 1  ridx=0
      settings: SourceProductBaseCode=SL
  Data Type Conversion : DataTypeConversion  OutDataTypeStr=DTsig_in  ConvertRealWorld=Stored Integer (SI)
  Real-Imag to Complex : RealImagToComplex
  Out1 : Outport
  wires:
  Bit Slice1/1 -> Real-Imag to Complex/2
  Bit Slice/1 -> Real-Imag to Complex/1
  Data Type Conversion/1 -> Out1/1
  Real-Imag to Complex/1 -> Data Type Conversion/1
  In1/1 -> Bit Slice1/1, Bit Slice/1

== system bramBurst_TransposeMatrix/PL DDR memory/DDR/Write Logic/Wr_control ==
  ddr_wr_rdy : Inport
  wr_enb : Inport  Port=2
  wr_len : Inport  Port=3
  AckGen : Subsystem
  MATLAB Function : MATLAB Function  TreatAsAtomicUnit=on
  Unit Delay : UnitDelay  SampleTime=-1  HasFrameUpgradeWarning=on
  valAddEnb : Outport  VectorParamsAs1DForOutWhenUnconnected=off
  axim_ack : Outport  Port=2  VectorParamsAs1DForOutWhenUnconnected=off
  ram_addr : Outport  Port=3  VectorParamsAs1DForOutWhenUnconnected=off
  wires:
  ddr_wr_rdy/1 -> AckGen/3(ddr_wr_rdy)
  AckGen/3(ram_addr) -> ram_addr/1
  Unit Delay/1 -> MATLAB Function/3(wr_ack), axim_ack/1
  MATLAB Function/1(wr_leng) -> AckGen/1(axiWrLen)
  AckGen/1(ack) -> Unit Delay/1
  wr_len/1 -> MATLAB Function/2(axi_wr_length)
  AckGen/2(ValAddEnb) -> valAddEnb/1
  wr_enb/1 -> MATLAB Function/1(axi_wr_en), AckGen/2(wrEnb)

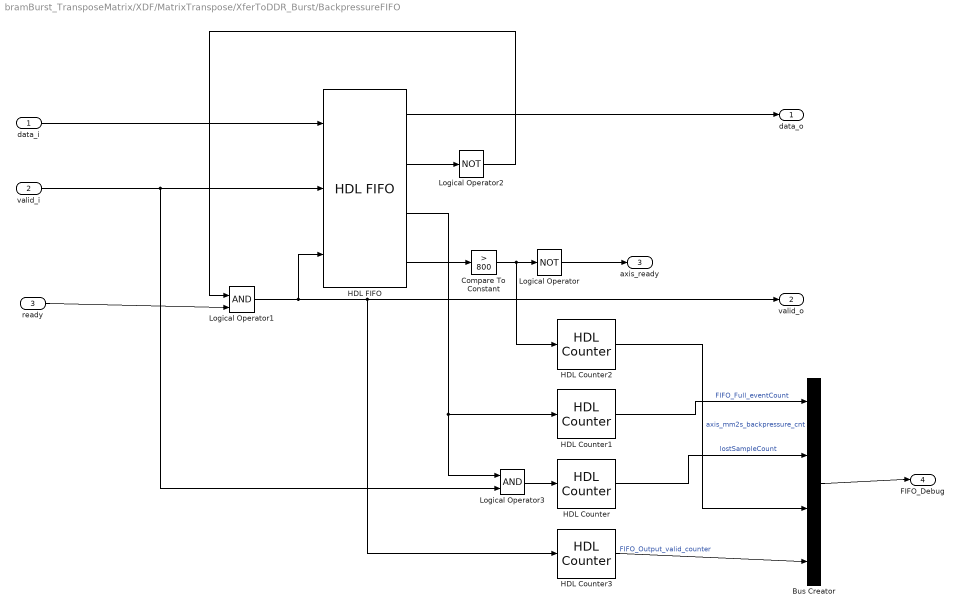
== system bramBurst_TransposeMatrix/XDF/MatrixTranspose/XferToDDR_Burst/BackpressureFIFO ==
  data_i : Inport
  valid_i : Inport  Port=2
  ready : Inport  Port=3
  Bus Creator : BusCreator  Inputs=4
  Compare To Constant : simulink/Logic and Bit Operations/Compare To Constant  relop=>  const=800  OutDataTypeStr=boolean
  HDL Counter{,1..3} (4 alike) : hdlsllib/Sources/HDL Counter  CountType=Free running  CountInit=0  CountStep=1  CountMax=25  CountFromType=Initial value  CountFrom=0  CountResetPort=off  CountLoadPort=off  CountEnbPort=on  CountDirPort=off  CountHitOutputPort=off  CountDataType=Unsigned  CountWordLen=32  CountFracLen=0  CountSampTime=1
  HDL FIFO : hdlsllib/HDL RAMs/HDL FIFO  fifo_size=1024  mode=FWFT  ratio=1  push_msg=Warning  pop_msg=Warning  show_empty=on  show_full=on  show_num=on  LabelModeActiveChoice_Mode=FWFT
      settings: SourceProductBaseCode=SL
  Logical Operator : Logic  Operator=NOT  IconShape=distinctive  AllPortsSameDT=off  OutDataTypeStr=boolean
  Logical Operator1 : Logic  IconShape=distinctive  AllPortsSameDT=off  OutDataTypeStr=boolean
  Logical Operator2 : Logic  Operator=NOT  IconShape=distinctive  AllPortsSameDT=off  OutDataTypeStr=boolean
  Logical Operator3 : Logic  AllPortsSameDT=off  OutDataTypeStr=boolean
  data_o : Outport
  valid_o : Outport  Port=2
  axis_ready : Outport  Port=3
  FIFO_Debug : Outport  Port=4
  wires:
  HDL FIFO/4 -> Compare To Constant/1
  HDL FIFO/2 -> Logical Operator2/1
  data_i/1 -> HDL FIFO/1
  Logical Operator1/1 -> HDL FIFO/3, HDL Counter3/1, valid_o/1
  HDL FIFO/1 -> data_o/1
  Logical Operator2/1 -> Logical Operator1/1
  Logical Operator/1 -> axis_ready/1
  Compare To Constant/1 -> HDL Counter2/1, Logical Operator/1
  valid_i/1 -> Logical Operator3/2, HDL FIFO/2
  ready/1 -> Logical Operator1/2
  HDL FIFO/3 -> Logical Operator3/1, HDL Counter1/1
  Logical Operator3/1 -> HDL Counter/1
  HDL Counter/1 -> Bus Creator/2  "lostSampleCount"
  HDL Counter1/1 -> Bus Creator/1  "FIFO_Full_eventCount"
  Bus Creator/1 -> FIFO_Debug/1
  HDL Counter2/1 -> Bus Creator/3  "axis_mm2s_backpressure_cnt"
  HDL Counter3/1 -> Bus Creator/4  "FIFO_Output_valid_counter"

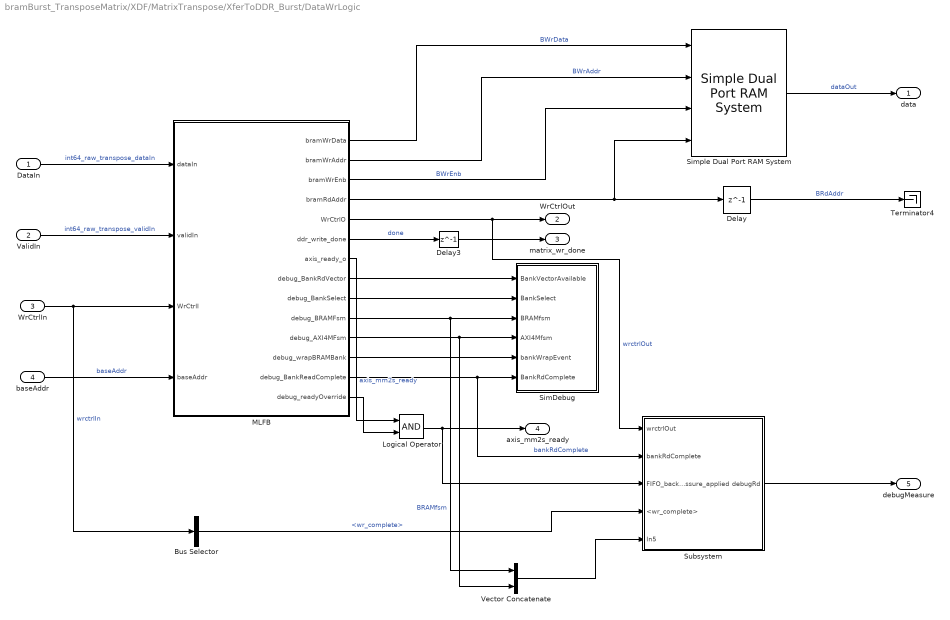
== system bramBurst_TransposeMatrix/XDF/MatrixTranspose/XferToDDR_Burst/DataWrLogic ==
  DataIn : Inport
  ValidIn : Inport  Port=2
  WrCtrlIn : Inport  Port=3
  baseAddr : Inport  Port=4
  Bus Selector : BusSelector  OutputSignals=wr_complete
  Delay : Delay  DelayLength=1
  Delay3 : Delay  DelayLength=1
  Logical Operator : Logic  AllPortsSameDT=off  OutDataTypeStr=boolean
  MLFB : MATLAB Function  TreatAsAtomicUnit=on  mask{pNumCols=hdlbramBurst.pNumCols, pNumRows=hdlbramBurst.pNumRows, pMaxBankLines=hdlbramBurst.pMaxBankLines, pMaxNumBanks=hdlbramBurst.pMaxNumBanks, pAXIDataWidthBytes=hdlbramBurst.pAXIDataWidthBytes, pBramAddrWidth=hdlbramBurst.pBramAddrWidth}
      mask prompts: pNumCols "Number of rows"; pNumRows "Number of col"; pMaxBankLines "Number of samples per line"; pMaxNumBanks "Number of banks"; pAXIDataWidthBytes "AXI4 data width in bytes"; pBramAddrWidth "BRAM Address Width"
  SimDebug : Subsystem
  Simple Dual Port RAM System : hdlsllib/HDL RAMs/Simple Dual Port RAM System  RAMType=Simple dual port  WriteOutputValue=New data  RAMInitialValue=0  SimulateUsing=Code generation
      settings: SourceProductBaseCode=SL
  Subsystem : Subsystem
  Terminator4 : Terminator
  Vector Concatenate : Concatenate
  data : Outport
  WrCtrlOut : Outport  Port=2
  matrix_wr_done : Outport  Port=3
  axis_mm2s_ready : Outport  Port=4
  debugMeasure : Outport  Port=5
  wires:
  MLFB/6(ddr_write_done) -> Delay3/1  "done"
  MLFB/5(WrCtrlO) -> Subsystem/1(wrctrlOut), WrCtrlOut/1  "wrctrlOut"
  Simple Dual Port RAM System/1 -> data/1  "dataOut"
  baseAddr/1 -> MLFB/4(baseAddr)  "baseAddr"
  WrCtrlIn/1 -> Bus Selector/1, MLFB/3(WrCtrlI)  "wrctrlIn"
  MLFB/1(bramWrData) -> Simple Dual Port RAM System/1  "BWrData"
  ValidIn/1 -> MLFB/2(validIn)  "int64_raw_transpose_validIn"
  DataIn/1 -> MLFB/1(dataIn)  "int64_raw_transpose_dataIn"
  MLFB/4(bramRdAddr) -> Simple Dual Port RAM System/4, Delay/1
  MLFB/2(bramWrAddr) -> Simple Dual Port RAM System/2  "BWrAddr"
  MLFB/3(bramWrEnb) -> Simple Dual Port RAM System/3  "BWrEnb"
  Delay3/1 -> matrix_wr_done/1
  Delay/1 -> Terminator4/1  "BRdAddr"
  MLFB/7(axis_ready_o) -> Logical Operator/1  "axis_mm2s_ready"
  MLFB/14(debug_readyOverride) -> Logical Operator/2
  Logical Operator/1 -> Subsystem/3(FIFO_backpressure_applied), axis_mm2s_ready/1
  MLFB/8(debug_BankRdVector) -> SimDebug/1(BankVectorAvailable)
  MLFB/9(debug_BankSelect) -> SimDebug/2(BankSelect)
  MLFB/10(debug_BRAMFsm) -> Vector Concatenate/1, SimDebug/3(BRAMfsm)  "BRAMfsm"
  MLFB/11(debug_AXI4MFsm) -> Vector Concatenate/2, SimDebug/4(AXI4Mfsm)
  MLFB/12(debug_wrapBRAMBank) -> SimDebug/5(bankWrapEvent)
  MLFB/13(debug_BankReadComplete) -> Subsystem/2(bankRdComplete), SimDebug/6(BankRdComplete)  "bankRdComplete"
  Bus Selector/1 -> Subsystem/4(<wr_complete>)  "<wr_complete>"
  Subsystem/1(debugRd) -> debugMeasure/1
  Vector Concatenate/1 -> Subsystem/5(In5)
